simulink model "MPC_resetable_THISONE"  (R2020b)
settings: Solver=VariableStepAuto  StartTime=0.0  StopTime=10  FixedStep=0.01  RelTol=1e-3
values from neighbouring files (symbols this model uses):
  A_2 = zeros(3)    [MPC_tune.m]
  B_2 = I_inv    [MPC_tune.m]
  C_2 = eye(3)    [MPC_tune.m]
  D_2 = zeros(3)    [MPC_tune.m]
  I_inv = inv(I_mat)    [MPC_tune.m]
undefined symbols (not defined in the file or in its folder): theta0
libraries: pid_lib x3, fuzblock x3, mpclib x1, dspmathops x1
settings Model: Creator=Jonathan van Zyl  LastModifiedBy=Jonathan van Zyl

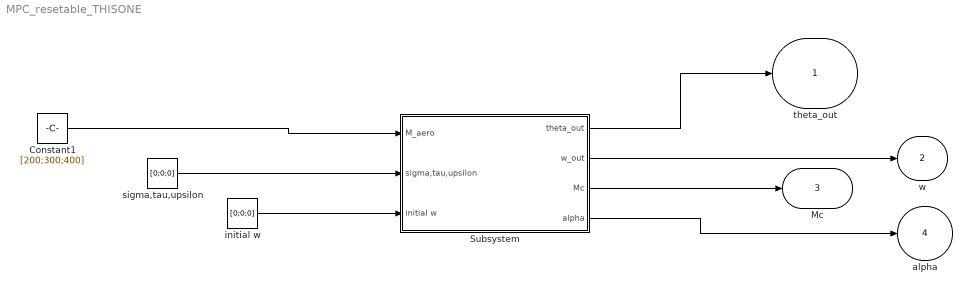
== system MPC_resetable_THISONE ==
  Constant1 : Constant  Value=[200;300;400]
  Subsystem : Subsystem
  initial w : Constant  Value=[0;0;0]
  sigma,tau,upsilon : Constant  Value=[0;0;0]
  theta_out : Outport
  w : Outport  Port=2
  Mc : Outport  Port=3
  alpha : Outport  Port=4
  wires:
  Constant1/1 -> Subsystem/1(M_aero)
  sigma,tau,upsilon/1 -> Subsystem/2(sigma,tau,upsilon)
  initial w/1 -> Subsystem/3(initial w)
  Subsystem/1(theta_out) -> theta_out/1
  Subsystem/2(w_out) -> w/1
  Subsystem/3(Mc) -> Mc/1
  Subsystem/4(alpha) -> alpha/1

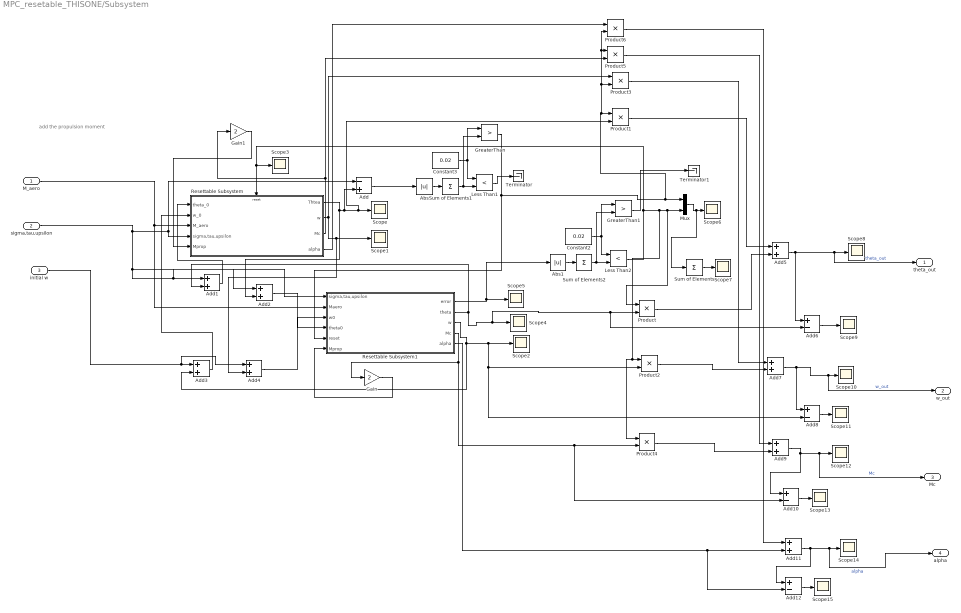
== system MPC_resetable_THISONE/Subsystem ==
  note: add the propulsion moment
  M_aero : Inport
  sigma,tau,upsilon : Inport  Port=2
  initial w : Inport  Port=3
  Abs : Abs
  Abs1 : Abs
  Add : Sum  Inputs=-+
  Add{1..5,7,9,11} (8 alike) : Sum
  Add{6,8,10,12} (4 alike) : Sum  Inputs=+-
  Constant2 : Constant  Value=0.02
  Constant3 : Constant  Value=0.02
  Gain : Gain  Gain=2
  Gain1 : Gain  Gain=2
  GreaterThan : RelationalOperator  Operator=>  OutDataTypeStr=boolean  RndMeth=Simplest
  GreaterThan1 : RelationalOperator  Operator=>  OutDataTypeStr=boolean  RndMeth=Simplest
  Less Than1 : RelationalOperator  Operator=<  OutDataTypeStr=boolean  RndMeth=Simplest
  Less Than2 : RelationalOperator  Operator=<  OutDataTypeStr=boolean  RndMeth=Simplest
  Mux : Mux  Inputs=2
  Product{,1..6} (7 alike) : Product
  Resettable Subsystem : Subsystem  TreatAsAtomicUnit=on
  Resettable Subsystem1 : Subsystem  TreatAsAtomicUnit=on
  Scope{,1..15} (16 alike) : Scope
  Sum of Elements : Sum  Inputs=+
  Sum of Elements1 : Sum  Inputs=+
  Sum of Elements2 : Sum  Inputs=+
  Terminator : Terminator
  Terminator1 : Terminator
  theta_out : Outport
  w_out : Outport  Port=2
  Mc : Outport  Port=3
  alpha : Outport  Port=4
  wires:
  Add8/1 -> Scope11/1
  GreaterThan/1 -> Product6/2, Product5/1, Product3/2, Product1/1, Mux/1, Resettable Subsystem1/5(reset)
  Add6/1 -> Scope9/1
  Abs1/1 -> Sum of Elements2/1
  Product1/1 -> Add5/1
  Resettable Subsystem/2(w) -> Scope1/1, Add4/2, Product3/1
  Resettable Subsystem1/4(Mc) -> Add10/2, Product4/2, Gain/1
  Resettable Subsystem1/2(theta) -> Add6/2, Product/2, Scope4/1, Add1/2
  Resettable Subsystem1/5(alpha) -> Add12/2, Add11/2
  Resettable Subsystem/1(Thtea) -> Add2/2, Add/2, Product1/2, Scope/1
  Less Than2/1 -> Product2/1, Product4/1, Product/1, Mux/2, Scope3/1, Resettable Subsystem/Reset
  M_aero/1 -> Resettable Subsystem1/2(Maero), Resettable Subsystem/3(M_aero)
  Resettable Subsystem1/1(error) -> Abs1/1, Scope5/1
  Add11/1 -> Add12/1, alpha/1, Scope14/1  "alpha"
  Product2/1 -> Add7/2
  Constant2/1 -> GreaterThan1/1, Less Than2/1
  Resettable Subsystem1/3(w) -> Add3/2, Scope2/1, Add8/2, Product2/2
  Product3/1 -> Add7/1
  Add12/1 -> Scope15/1
  Abs/1 -> Sum of Elements1/1
  Add5/1 -> Add6/1, theta_out/1, Scope8/1  "theta_out"
  Add2/1 -> Resettable Subsystem1/4(theta0)
  Constant3/1 -> GreaterThan/1, Less Than1/1
  Sum of Elements1/1 -> Less Than1/2, GreaterThan/2
  Add3/1 -> Resettable Subsystem/2(w_0)
  sigma,tau,upsilon/1 -> Add2/1, Add1/1, Resettable Subsystem1/1(sigma,tau,upsilon), Add/1, Resettable Subsystem/4(sigma,tau,upsilon)
  Product5/1 -> Add9/1
  Resettable Subsystem/3(Mc) -> Product5/2, Gain1/1
  Add7/1 -> Add8/1, w_out/1, Scope10/1  "w_out"
  Product6/1 -> Add11/1
  Add9/1 -> Add10/1, Mc/1, Scope12/1  "Mc"
  Add/1 -> Abs/1
  Add1/1 -> Resettable Subsystem/1(theta_0)
  Sum of Elements/1 -> Scope7/1
  Gain/1 -> Resettable Subsystem1/6(Mprop)
  Sum of Elements2/1 -> Less Than2/2, GreaterThan1/2
  Gain1/1 -> Resettable Subsystem/5(Mprop)
  Mux/1 -> Sum of Elements/1, Scope6/1
  Resettable Subsystem/4(alpha) -> Product6/1
  Add4/1 -> Resettable Subsystem1/3(w0)
  initial w/1 -> Add4/1, Add3/1
  Product/1 -> Add5/2
  Add10/1 -> Scope13/1
  Product4/1 -> Add9/2
  GreaterThan1/1 -> Terminator1/1
  Less Than1/1 -> Terminator/1

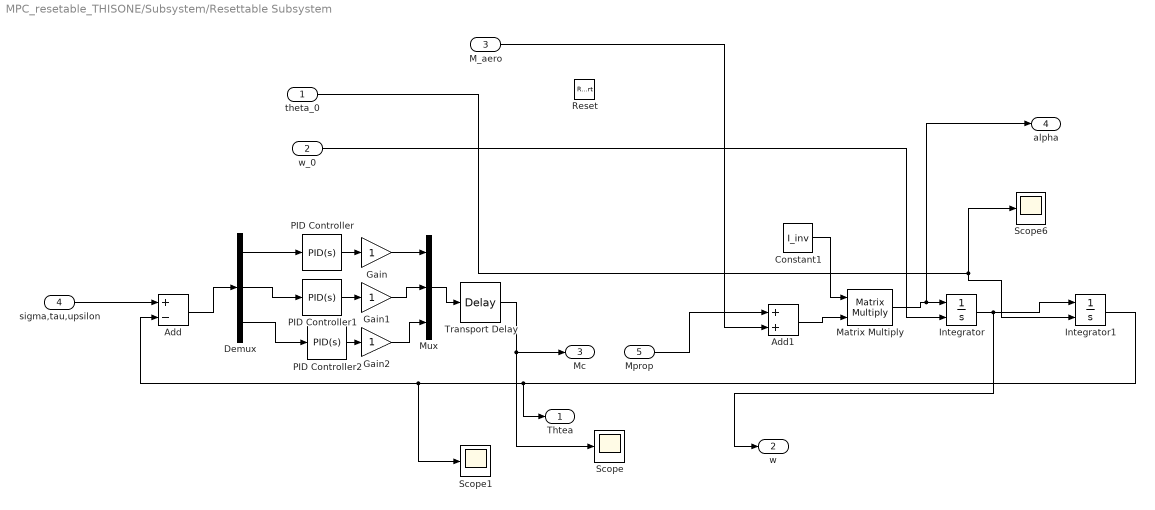
== system MPC_resetable_THISONE/Subsystem/Resettable Subsystem ==
  theta_0 : Inport
  w_0 : Inport  Port=2
  M_aero : Inport  Port=3
  sigma,tau,upsilon : Inport  Port=4
  Mprop : Inport  Port=5
  Reset : ResetPort  DisableCoverage=on  ResetTriggerType=either
  Add : Sum  Inputs=+-
  Add1 : Sum
  Constant1 : Constant  Value=I_inv
  Demux : Demux  Outputs=3
  Gain : Gain
  Gain1 : Gain
  Gain2 : Gain
  Integrator : Integrator  InitialConditionSource=external  InitialCondition=[0.15;-0.2;0.01]
  Integrator1 : Integrator  InitialConditionSource=external  InitialCondition=[0.01;-0.01;0.005]
  Matrix Multiply : Product  Multiplication=Matrix(*)
  Mux : Mux  Inputs=3
  PID Controller : pid_lib/PID Controller  Controller=PID  Form=Parallel  TimeDomain=Continuous-time  UseExternalTs=off  SampleTime=-1  IntegratorMethod=Forward Euler  FilterMethod=Forward Euler  ControllerParametersSource=internal  P=76.4274415550338  I=3.57793373088927  D=400.875615235633  UseFilter=on  N=5.45397025421619  TunerSelectOption=Transfer Function Based (PID Tuner App)  InitialConditionSource=internal  InitialConditionForIntegrator=0  InitialConditionForFilter=0  DifferentiatorICPrevScaledInput=0  ExternalReset=none  TrackingMode=off  Kt=1  LimitOutput=off  SatLimitsSource=internal  UpperSaturationLimit=inf  LowerSaturationLimit=-inf  LinearizeAsGain=on  AntiWindupMode=none  Kb=1  POutMin=[]  POutMax=[]  IOutMin=[]  IOutMax=[]  DOutMin=[]  DOutMax=[]  NOutMin=[]  NOutMax=[]  SumOutMin=[]  SumOutMax=[]  SaturationOutMin=[]  SaturationOutMax=[]  PParamMin=[]  PParamMax=[]  IParamMin=[]  IParamMax=[]  DParamMin=[]  DParamMax=[]  NParamMin=[]  NParamMax=[]  KbParamMin=[]  KbParamMax=[]  KtParamMin=[]  KtParamMax=[]  KbOutMin=[]  KbOutMax=[]  KtOutMin=[]  KtOutMax=[]  IntegratorOutMin=[]  IntegratorOutMax=[]  FilterOutMin=[]  FilterOutMax=[]  SumI1OutMin=[]  SumI1OutMax=[]  SumI2OutMin=[]  SumI2OutMax=[]  SumI3OutMin=[]  SumI3OutMax=[]  SumI4OutMin=[]  SumI4OutMax=[]  SumDOutMin=[]  SumDOutMax=[]  DifferentiatorOutMin=[]  DifferentiatorOutMax=[]  FilterDiffOutCoefMin=[]  FilterDiffOutCoefMax=[]  ReciprocalOutMin=[]  ReciprocalOutMax=[]  SumDenOutMin=[]  SumDenOutMax=[]  SumNumOutMin=[]  SumNumOutMax=[]  DivideOutMin=[]  DivideOutMax=[]  UdiffTsProdOutMin=[]  UdiffTsProdOutMax=[]  NTsProdOutMin=[]  NTsProdOutMax=[]  UintegralTsProdOutMin=[]  UintegralTsProdOutMax=[]  UngainTsProdOutMin=[]  UngainTsProdOutMax=[]  IntegratorContinuousStateAttributes=''  IntegratorStateMustResolveToSignalObject=off  IntegratorRTWStateStorageClass=Auto  FilterContinuousStateAttributes=''  FilterStateMustResolveToSignalObject=off  FilterRTWStateStorageClass=Auto  ParallelPVariant=InternalParameters  IdealPVariant=Disabled  IVariant=InternalParameters  DVariant=InternalParameters  IntegratorVariant=Continuous  SatVariant=Disabled  AWVariant=Passthrough  PCopyVariant=Disabled  TRVariant=Disabled  FdbkBlocksVariant=Forward  IdealPFdbkVariant=Disabled  SatFdbkVariant=Disabled  DerivativeFilterVariant=ContFilter  NVariant=InternalParameters  NCopyVariant=Disabled  FilterICVariant=InternalICsFilter  IntegratorICVariant=InternalICs  ExternalResetVariant=Disabled  TRSumVariant=Passthrough  SumFdbkVariant=Disabled  SumVariant=Sum_PID  TsampFilterVariant=InternalTs  TsampNgainVariant=Passthrough  TsampIntegralVariant=Passthrough  ExternalSaturationOutDataTypeStr=Inherit: Same as second input
  PID Controller1 : pid_lib/PID Controller  Controller=PID  Form=Parallel  TimeDomain=Continuous-time  UseExternalTs=off  SampleTime=-1  IntegratorMethod=Forward Euler  FilterMethod=Forward Euler  ControllerParametersSource=internal  P=-202.527799620363  I=-9.48129403471772  D=-1062.29457146841  UseFilter=on  N=5.45397025421619  TunerSelectOption=Transfer Function Based (PID Tuner App)  InitialConditionSource=internal  InitialConditionForIntegrator=0  InitialConditionForFilter=0  DifferentiatorICPrevScaledInput=0  ExternalReset=none  TrackingMode=off  Kt=1  LimitOutput=off  SatLimitsSource=internal  UpperSaturationLimit=inf  LowerSaturationLimit=-inf  LinearizeAsGain=on  AntiWindupMode=none  Kb=1  POutMin=[]  POutMax=[]  IOutMin=[]  IOutMax=[]  DOutMin=[]  DOutMax=[]  NOutMin=[]  NOutMax=[]  SumOutMin=[]  SumOutMax=[]  SaturationOutMin=[]  SaturationOutMax=[]  PParamMin=[]  PParamMax=[]  IParamMin=[]  IParamMax=[]  DParamMin=[]  DParamMax=[]  NParamMin=[]  NParamMax=[]  KbParamMin=[]  KbParamMax=[]  KtParamMin=[]  KtParamMax=[]  KbOutMin=[]  KbOutMax=[]  KtOutMin=[]  KtOutMax=[]  IntegratorOutMin=[]  IntegratorOutMax=[]  FilterOutMin=[]  FilterOutMax=[]  SumI1OutMin=[]  SumI1OutMax=[]  SumI2OutMin=[]  SumI2OutMax=[]  SumI3OutMin=[]  SumI3OutMax=[]  SumI4OutMin=[]  SumI4OutMax=[]  SumDOutMin=[]  SumDOutMax=[]  DifferentiatorOutMin=[]  DifferentiatorOutMax=[]  FilterDiffOutCoefMin=[]  FilterDiffOutCoefMax=[]  ReciprocalOutMin=[]  ReciprocalOutMax=[]  SumDenOutMin=[]  SumDenOutMax=[]  SumNumOutMin=[]  SumNumOutMax=[]  DivideOutMin=[]  DivideOutMax=[]  UdiffTsProdOutMin=[]  UdiffTsProdOutMax=[]  NTsProdOutMin=[]  NTsProdOutMax=[]  UintegralTsProdOutMin=[]  UintegralTsProdOutMax=[]  UngainTsProdOutMin=[]  UngainTsProdOutMax=[]  IntegratorContinuousStateAttributes=''  IntegratorStateMustResolveToSignalObject=off  IntegratorRTWStateStorageClass=Auto  FilterContinuousStateAttributes=''  FilterStateMustResolveToSignalObject=off  FilterRTWStateStorageClass=Auto  ParallelPVariant=InternalParameters  IdealPVariant=Disabled  IVariant=InternalParameters  DVariant=InternalParameters  IntegratorVariant=Continuous  SatVariant=Disabled  AWVariant=Passthrough  PCopyVariant=Disabled  TRVariant=Disabled  FdbkBlocksVariant=Forward  IdealPFdbkVariant=Disabled  SatFdbkVariant=Disabled  DerivativeFilterVariant=ContFilter  NVariant=InternalParameters  NCopyVariant=Disabled  FilterICVariant=InternalICsFilter  IntegratorICVariant=InternalICs  ExternalResetVariant=Disabled  TRSumVariant=Passthrough  SumFdbkVariant=Disabled  SumVariant=Sum_PID  TsampFilterVariant=InternalTs  TsampNgainVariant=Passthrough  TsampIntegralVariant=Passthrough  ExternalSaturationOutDataTypeStr=Inherit: Same as second input
  PID Controller2 : pid_lib/PID Controller  Controller=PID  Form=Parallel  TimeDomain=Continuous-time  UseExternalTs=off  SampleTime=-1  IntegratorMethod=Forward Euler  FilterMethod=Forward Euler  ControllerParametersSource=internal  P=-232.294042315359  I=-10.8747940867059  D=-1218.42384402842  UseFilter=on  N=5.45397025421619  TunerSelectOption=Transfer Function Based (PID Tuner App)  InitialConditionSource=internal  InitialConditionForIntegrator=0  InitialConditionForFilter=0  DifferentiatorICPrevScaledInput=0  ExternalReset=none  TrackingMode=off  Kt=1  LimitOutput=off  SatLimitsSource=internal  UpperSaturationLimit=inf  LowerSaturationLimit=-inf  LinearizeAsGain=on  AntiWindupMode=none  Kb=1  POutMin=[]  POutMax=[]  IOutMin=[]  IOutMax=[]  DOutMin=[]  DOutMax=[]  NOutMin=[]  NOutMax=[]  SumOutMin=[]  SumOutMax=[]  SaturationOutMin=[]  SaturationOutMax=[]  PParamMin=[]  PParamMax=[]  IParamMin=[]  IParamMax=[]  DParamMin=[]  DParamMax=[]  NParamMin=[]  NParamMax=[]  KbParamMin=[]  KbParamMax=[]  KtParamMin=[]  KtParamMax=[]  KbOutMin=[]  KbOutMax=[]  KtOutMin=[]  KtOutMax=[]  IntegratorOutMin=[]  IntegratorOutMax=[]  FilterOutMin=[]  FilterOutMax=[]  SumI1OutMin=[]  SumI1OutMax=[]  SumI2OutMin=[]  SumI2OutMax=[]  SumI3OutMin=[]  SumI3OutMax=[]  SumI4OutMin=[]  SumI4OutMax=[]  SumDOutMin=[]  SumDOutMax=[]  DifferentiatorOutMin=[]  DifferentiatorOutMax=[]  FilterDiffOutCoefMin=[]  FilterDiffOutCoefMax=[]  ReciprocalOutMin=[]  ReciprocalOutMax=[]  SumDenOutMin=[]  SumDenOutMax=[]  SumNumOutMin=[]  SumNumOutMax=[]  DivideOutMin=[]  DivideOutMax=[]  UdiffTsProdOutMin=[]  UdiffTsProdOutMax=[]  NTsProdOutMin=[]  NTsProdOutMax=[]  UintegralTsProdOutMin=[]  UintegralTsProdOutMax=[]  UngainTsProdOutMin=[]  UngainTsProdOutMax=[]  IntegratorContinuousStateAttributes=''  IntegratorStateMustResolveToSignalObject=off  IntegratorRTWStateStorageClass=Auto  FilterContinuousStateAttributes=''  FilterStateMustResolveToSignalObject=off  FilterRTWStateStorageClass=Auto  ParallelPVariant=InternalParameters  IdealPVariant=Disabled  IVariant=InternalParameters  DVariant=InternalParameters  IntegratorVariant=Continuous  SatVariant=Disabled  AWVariant=Passthrough  PCopyVariant=Disabled  TRVariant=Disabled  FdbkBlocksVariant=Forward  IdealPFdbkVariant=Disabled  SatFdbkVariant=Disabled  DerivativeFilterVariant=ContFilter  NVariant=InternalParameters  NCopyVariant=Disabled  FilterICVariant=InternalICsFilter  IntegratorICVariant=InternalICs  ExternalResetVariant=Disabled  TRSumVariant=Passthrough  SumFdbkVariant=Disabled  SumVariant=Sum_PID  TsampFilterVariant=InternalTs  TsampNgainVariant=Passthrough  TsampIntegralVariant=Passthrough  ExternalSaturationOutDataTypeStr=Inherit: Same as second input
  Scope : Scope
  Scope1 : Scope
  Scope6 : Scope
  Transport Delay : TransportDelay  DelayTime=0.1
  Thtea : Outport
  w : Outport  Port=2
  Mc : Outport  Port=3
  alpha : Outport  Port=4
  wires:
  Transport Delay/1 -> Mc/1, Scope/1
  Constant1/1 -> Matrix Multiply/1
  PID Controller2/1 -> Gain2/1
  PID Controller/1 -> Gain/1
  Matrix Multiply/1 -> alpha/1, Integrator/1
  Demux/3 -> PID Controller2/1
  Mux/1 -> Transport Delay/1
  sigma,tau,upsilon/1 -> Add/1
  Gain/1 -> Mux/1
  w_0/1 -> Integrator/2
  Gain2/1 -> Mux/3
  Add/1 -> Demux/1
  Add1/1 -> Matrix Multiply/2
  PID Controller1/1 -> Gain1/1
  Integrator/1 -> w/1, Integrator1/1
  theta_0/1 -> Integrator1/2, Scope6/1
  Demux/2 -> PID Controller1/1
  Gain1/1 -> Mux/2
  M_aero/1 -> Add1/2
  Demux/1 -> PID Controller/1
  Integrator1/1 -> Thtea/1, Scope1/1, Add/2
  Mprop/1 -> Add1/1

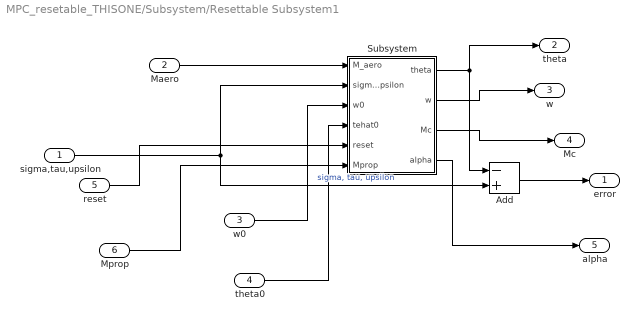
== system MPC_resetable_THISONE/Subsystem/Resettable Subsystem1 ==
  sigma,tau,upsilon : Inport
  Maero : Inport  Port=2
  w0 : Inport  Port=3
  theta0 : Inport  Port=4
  reset : Inport  Port=5
  Mprop : Inport  Port=6
  Add : Sum  Inputs=-+
  Subsystem : Subsystem
  error : Outport
  theta : Outport  Port=2
  w : Outport  Port=3
  Mc : Outport  Port=4
  alpha : Outport  Port=5
  wires:
  theta0/1 -> Subsystem/4(tehat0)
  Subsystem/2(w) -> w/1
  Add/1 -> error/1
  Maero/1 -> Subsystem/1(M_aero)
  sigma,tau,upsilon/1 -> Add/2, Subsystem/2(sigma,tau,upsilon)  "sigma, tau, upsilon"
  Subsystem/1(theta) -> Add/1, theta/1
  w0/1 -> Subsystem/3(w0)
  reset/1 -> Subsystem/5(reset)
  Subsystem/3(Mc) -> Mc/1
  Mprop/1 -> Subsystem/6(Mprop)
  Subsystem/4(alpha) -> alpha/1

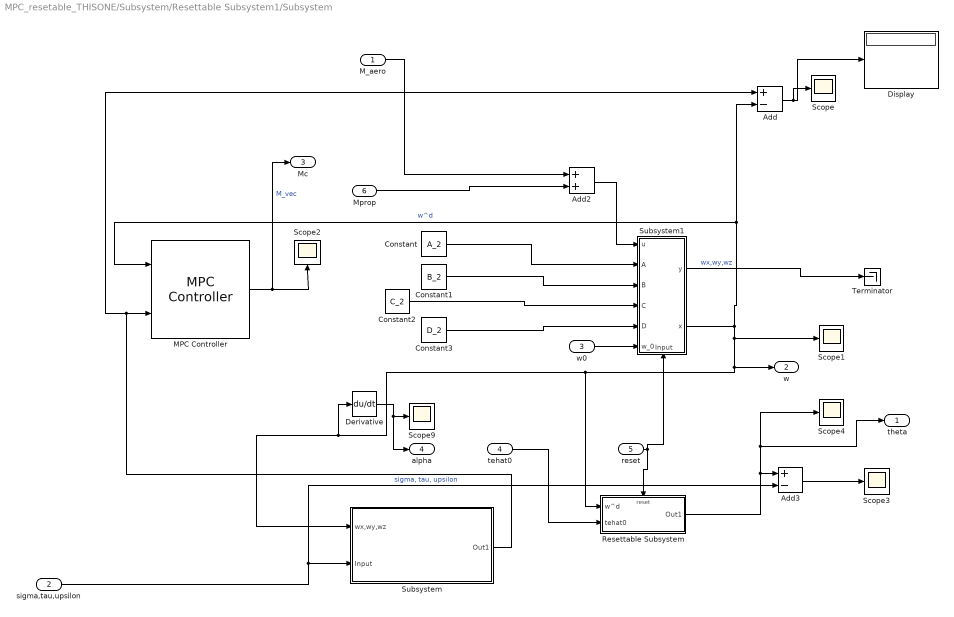
== system MPC_resetable_THISONE/Subsystem/Resettable Subsystem1/Subsystem ==
  M_aero : Inport
  sigma,tau,upsilon : Inport  Port=2
  w0 : Inport  Port=3
  tehat0 : Inport  Port=4
  reset : Inport  Port=5
  Mprop : Inport  Port=6
  Add : Sum  Inputs=+-
  Add2 : Sum
  Add3 : Sum  Inputs=+-
  Constant : Constant  Value=A_2
  Constant1 : Constant  Value=B_2
  Constant2 : Constant  Value=C_2
  Constant3 : Constant  Value=D_2
  Derivative : Derivative
  Display : Display
  MPC Controller : mpclib/MPC Controller  SCDEnableBlockLinearizationSpecification=on  mpcobj=MPCDesignerSession.AppData.Controllers.MPC  is_multiple=0  enable_value=0  return_u0=off  updateMPCinCallerWorkspace=on  md_inport=off  mv_inport=off  uref_inport=off  return_cost=off  return_mvseq=off  return_qpstatus=off  return_xseq=off  return_state=off  return_ovseq=off  state_inport=off  umin_inport=off  umax_inport=off  ymin_inport=off  ymax_inport=off  cc_inport=off  ywt_inport=off  uwt_inport=off  duwt_inport=off  rhoeps_inport=off  pm_inport=off  MaximumP=10  HorizonChoice=FixedHorizon  n_ts=0.1  n_p=10  n_mv=3  n_md=0  n_ud=0  n_mo=3  n_uo=0  BlockDataType=double  SampleTimeInherited=off  switch_inport=off
  Resettable Subsystem : Subsystem  TreatAsAtomicUnit=on
  Scope{,1..4,9} (6 alike) : Scope
  Subsystem : Subsystem
  Subsystem1 : Subsystem
      settings: PortSchema="{\"entries\":[{\"content\":{\"sides\":[{\"content\":{\"connectorIds\":[\"In1\",\"In2\",\"In3\",\"In4\",\"In5\",\"In6\"]},\"type\":\"ConnectorPlacement.EquallySpacedRectSide\",\"uuid\":\"7d9460a7-3adf-4f89-91e7-b456f7078c86\"},{\"content\":{\"connectorIds\":[\"Out1\",\"Out2\"],\"side\":\"RIGHT\"},\"type\":\"ConnectorPlacement.EquallySpacedRectSide\",\"uuid\":\"f1bf29ac-ed67-4ce4-91e2-85f2b90efa08\"},{\"content\":{\"connectorIds\":[],\"side\":\"TOP\"},\"type\":\"ConnectorPlacement.EquallySpacedRectSide\",\"uuid\":\"d922c634-a6d8-424b-a167-3b858780e5fe\"},{\"content\":{\"connectorIds\":[\"In7\"],\"side\":\"BOTTOM\"},\"type\":\"ConnectorPlacement.EquallySpacedRectSide\",\"uuid\":\"f177f641-1570-409d-a38e-cef2b78f705f\"},{\"content\":{\"connectorIds\":[],\"side\":\"HIDDEN\"},\"type\":\"ConnectorPlacement.EquallySpacedRectSide\",\"uuid\":\"30cf80c6-7b26-40df-a778-919a6a544dd2\"}]},\"type\":\"ConnectorPlacement.EquallySpacedConnector\",\"uuid\":\"27252b95-3211-4624-87a6-4be9d32d6c6a\"}],\"packageUris\":[\"http://schema.mathworks.com/mf0/Connector/R2020b\"],\"version\":\"1.0\"}"
  Terminator : Terminator
  theta : Outport
  w : Outport  Port=2
  Mc : Outport  Port=3
  alpha : Outport  Port=4
  wires:
  Subsystem1/1(y) -> Terminator/1  "wx,wy,wz"
  Derivative/1 -> alpha/1, Scope9/1
  Resettable Subsystem/1(Out1) -> Scope4/1, theta/1, Add3/1
  Add/1 -> Display/1, Scope/1
  Add3/1 -> Scope3/1
  Add2/1 -> Subsystem1/1(u)
  sigma,tau,upsilon/1 -> Add3/2, Subsystem/2(Input)  "sigma, tau, upsilon"
  Subsystem/1(Out1) -> Add/1, MPC Controller/2
  M_aero/1 -> Add2/1
  Constant2/1 -> Subsystem1/4(C)
  Constant3/1 -> Subsystem1/5(D)
  Subsystem1/2(x) -> Add/2, MPC Controller/1, Scope1/1, w/1, Resettable Subsystem/1(w^d), Subsystem/1(wx,wy,wz), Derivative/1  "w^d"
  MPC Controller/1 -> Mc/1, Scope2/1  "M_vec"
  Constant/1 -> Subsystem1/2(A)
  Constant1/1 -> Subsystem1/3(B)
  w0/1 -> Subsystem1/6(w_0)
  tehat0/1 -> Resettable Subsystem/2(tehat0)
  reset/1 -> Subsystem1/7(Input), Resettable Subsystem/Reset
  Mprop/1 -> Add2/2

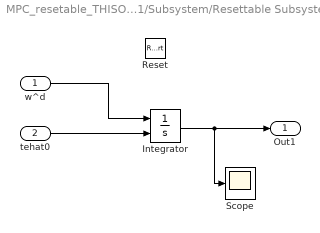
== system MPC_resetable_THISONE/Subsystem/Resettable Subsystem1/Subsystem/Resettable Subsystem ==
  w^d : Inport
  tehat0 : Inport  Port=2
  Reset : ResetPort  DisableCoverage=on
  Integrator : Integrator  InitialConditionSource=external  InitialCondition=theta0
  Scope : Scope
  Out1 : Outport
  wires:
  tehat0/1 -> Integrator/2
  w^d/1 -> Integrator/1
  Integrator/1 -> Scope/1, Out1/1

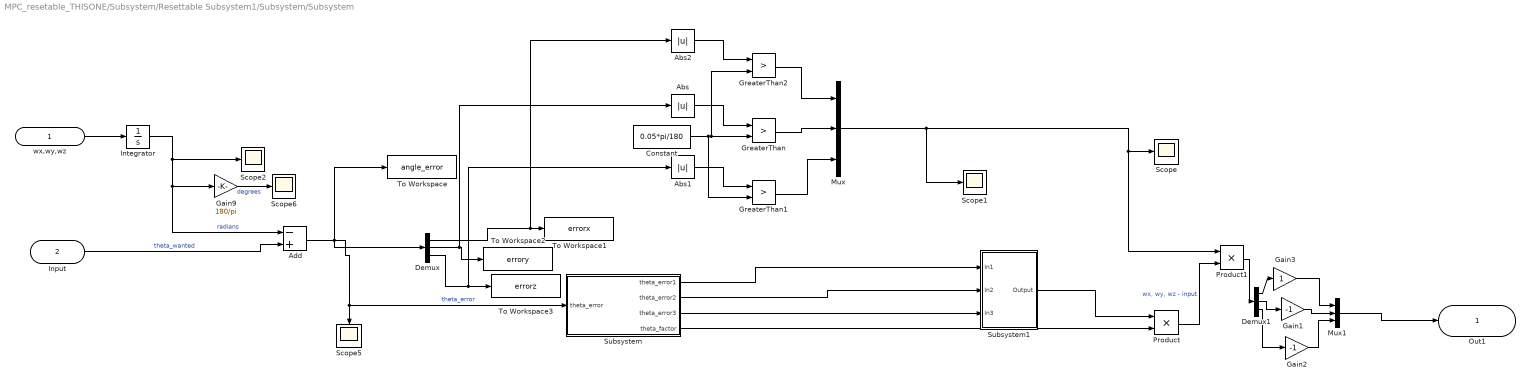
== system MPC_resetable_THISONE/Subsystem/Resettable Subsystem1/Subsystem/Subsystem ==
  wx,wy,wz : Inport
  Input : Inport  Port=2
  Abs : Abs
  Abs1 : Abs
  Abs2 : Abs
  Add : Sum  Inputs=-+
  Constant : Constant  Value=0.05*pi/180
  Demux : Demux  Outputs=3
  Demux1 : Demux  Outputs=3
  Gain1 : Gain  Gain=-1
  Gain2 : Gain  Gain=-1
  Gain3 : Gain
  Gain9 : Gain  Gain=180/pi
  GreaterThan : RelationalOperator  Operator=>  OutDataTypeStr=boolean  RndMeth=Simplest
  GreaterThan1 : RelationalOperator  Operator=>  OutDataTypeStr=boolean  RndMeth=Simplest
  GreaterThan2 : RelationalOperator  Operator=>  OutDataTypeStr=boolean  RndMeth=Simplest
  Integrator : Integrator  InitialCondition=[0;0;0]
  Mux : Mux  Inputs=3
  Mux1 : Mux  Inputs=3
  Product : Product
  Product1 : Product
  Scope{,1..2,5..6} (5 alike) : Scope
  Subsystem : Subsystem
  Subsystem1 : Subsystem
  To Workspace : ToWorkspace  VariableName=angle_error  SampleTime=-1
  To Workspace1 : ToWorkspace  VariableName=errorx  SaveFormat=Timeseries  SampleTime=-1
      settings: Save2DSignal=2-D array (concatenate along first dimension)
  To Workspace2 : ToWorkspace  VariableName=errory  SaveFormat=Timeseries  SampleTime=-1
  To Workspace3 : ToWorkspace  VariableName=errorz  SaveFormat=Timeseries  SampleTime=-1
  Out1 : Outport
  wires:
  Integrator/1 -> Add/1, Gain9/1, Scope2/1  "radians"
  Add/1 -> To Workspace/1, Demux/1, Subsystem/1(theta_error), Scope5/1  "theta_error"
  Gain9/1 -> Scope6/1  "degrees"
  Input/1 -> Add/2  "theta_wanted"
  Product/1 -> Product1/2  "wx, wy, wz - input"
  wx,wy,wz/1 -> Integrator/1
  Subsystem/4(theta_factor) -> Product/2
  Demux/2 -> Abs/1, To Workspace2/1
  Demux/3 -> Abs1/1, To Workspace3/1
  Demux/1 -> Abs2/1, To Workspace1/1
  Subsystem/1(theta_error1) -> Subsystem1/1(In1)
  Subsystem/2(theta_error2) -> Subsystem1/2(In2)
  Subsystem/3(theta_error3) -> Subsystem1/3(In3)
  Subsystem1/1(Output) -> Product/1
  Abs/1 -> GreaterThan/1
  Constant/1 -> GreaterThan1/2, GreaterThan2/2, GreaterThan/2
  Abs1/1 -> GreaterThan1/1
  Abs2/1 -> GreaterThan2/1
  GreaterThan2/1 -> Mux/1
  GreaterThan/1 -> Mux/2
  GreaterThan1/1 -> Mux/3
  Mux/1 -> Scope1/1, Scope/1, Product1/1
  Product1/1 -> Demux1/1
  Mux1/1 -> Out1/1
  Demux1/2 -> Gain1/1
  Demux1/3 -> Gain2/1
  Demux1/1 -> Gain3/1
  Gain3/1 -> Mux1/1
  Gain1/1 -> Mux1/2
  Gain2/1 -> Mux1/3

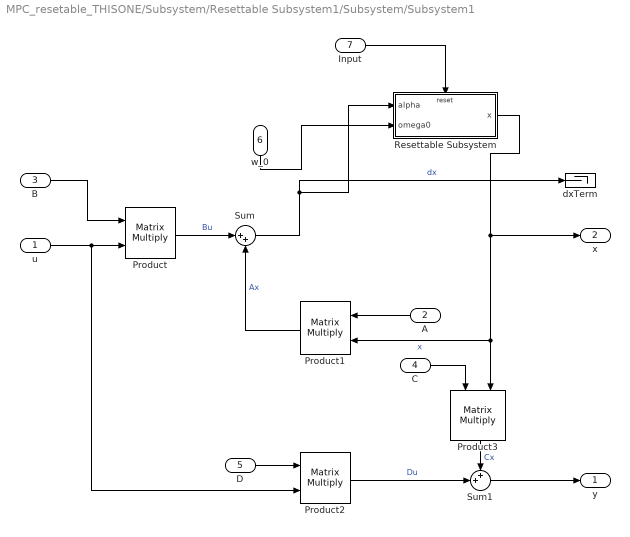
== system MPC_resetable_THISONE/Subsystem/Resettable Subsystem1/Subsystem/Subsystem1 ==
  u : Inport
  A : Inport  Port=2
  B : Inport  Port=3
  C : Inport  Port=4
  D : Inport  Port=5
  w_0 : Inport  Port=6
  Input : Inport  Port=7
  Product{,1..3} (4 alike) : Product  SCDEnableBlockLinearizationSpecification=on  Multiplication=Matrix(*)
  Resettable Subsystem : Subsystem  TreatAsAtomicUnit=on
  Sum : Sum  Inputs=|++
  Sum1 : Sum  Inputs=++|
  dxTerm : Terminator
  y : Outport  VectorParamsAs1DForOutWhenUnconnected=off
  x : Outport  Port=2  VectorParamsAs1DForOutWhenUnconnected=off
  wires:
  Sum/1 -> Resettable Subsystem/1(alpha), dxTerm/1  "dx"
  Product3/1 -> Sum1/1  "Cx"
  Product/1 -> Sum/1  "Bu"
  u/1 -> Product2/2, Product/2
  Product2/1 -> Sum1/2  "Du"
  Resettable Subsystem/1(x) -> x/1, Product1/2, Product3/2  "x"
  A/1 -> Product1/1
  Product1/1 -> Sum/2  "Ax"
  C/1 -> Product3/1
  B/1 -> Product/1
  D/1 -> Product2/1
  Sum1/1 -> y/1
  w_0/1 -> Resettable Subsystem/2(omega0)
  Input/1 -> Resettable Subsystem/Reset

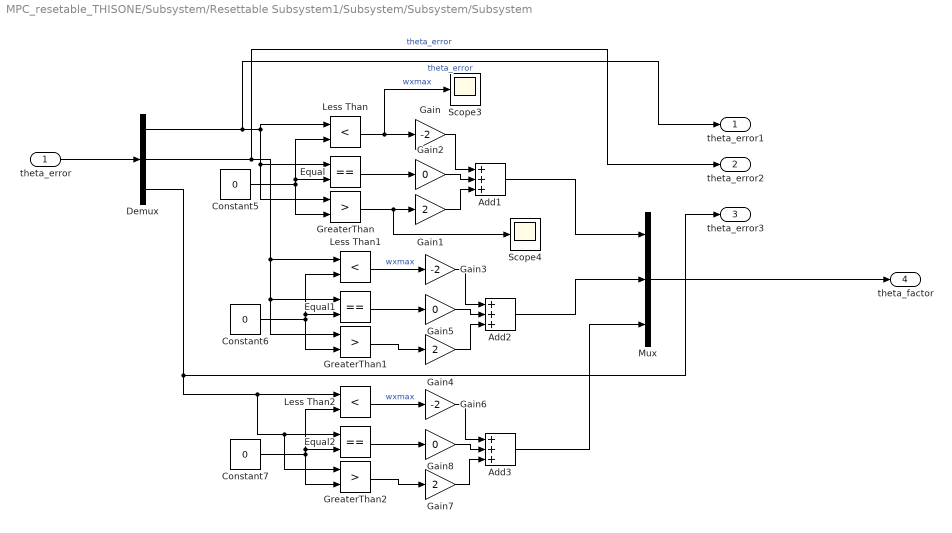
== system MPC_resetable_THISONE/Subsystem/Resettable Subsystem1/Subsystem/Subsystem/Subsystem ==
  theta_error : Inport
  Add1 : Sum  Inputs=+++
  Add2 : Sum  Inputs=+++
  Add3 : Sum  Inputs=+++
  Constant5 : Constant  Value=0
  Constant6 : Constant  Value=0
  Constant7 : Constant  Value=0
  Demux : Demux  Outputs=3
  Equal : RelationalOperator  Operator===  OutDataTypeStr=boolean  RndMeth=Simplest
  Equal1 : RelationalOperator  Operator===  OutDataTypeStr=boolean  RndMeth=Simplest
  Equal2 : RelationalOperator  Operator===  OutDataTypeStr=boolean  RndMeth=Simplest
  Gain : Gain  Gain=-2
  Gain1 : Gain  Gain=2
  Gain2 : Gain  Gain=0
  Gain3 : Gain  Gain=-2
  Gain4 : Gain  Gain=2
  Gain5 : Gain  Gain=0
  Gain6 : Gain  Gain=-2
  Gain7 : Gain  Gain=2
  Gain8 : Gain  Gain=0
  GreaterThan : RelationalOperator  Operator=>  OutDataTypeStr=boolean  RndMeth=Simplest
  GreaterThan1 : RelationalOperator  Operator=>  OutDataTypeStr=boolean  RndMeth=Simplest
  GreaterThan2 : RelationalOperator  Operator=>  OutDataTypeStr=boolean  RndMeth=Simplest
  Less Than : RelationalOperator  Operator=<  OutDataTypeStr=boolean  RndMeth=Simplest
  Less Than1 : RelationalOperator  Operator=<  OutDataTypeStr=boolean  RndMeth=Simplest
  Less Than2 : RelationalOperator  Operator=<  OutDataTypeStr=boolean  RndMeth=Simplest
  Mux : Mux  Inputs=3
  Scope3 : Scope
  Scope4 : Scope
  theta_error1 : Outport
  theta_error2 : Outport  Port=2
  theta_error3 : Outport  Port=3
  theta_factor : Outport  Port=4
  wires:
  Add1/1 -> Mux/1
  Constant5/1 -> Equal/2, Less Than/2, GreaterThan/2
  Equal2/1 -> Gain8/1
  Demux/1 -> theta_error1/1, GreaterThan/1, Equal/1, Less Than/1  "theta_error"
  GreaterThan2/1 -> Gain7/1
  Gain1/1 -> Add1/3
  Gain7/1 -> Add3/3
  Less Than1/1 -> Gain3/1  "wxmax"
  Gain6/1 -> Add3/1
  Equal/1 -> Gain2/1
  Gain5/1 -> Add2/2
  Add3/1 -> Mux/3
  GreaterThan/1 -> Scope4/1, Gain1/1
  Constant6/1 -> Equal1/2, Less Than1/2, GreaterThan1/2
  Demux/3 -> theta_error3/1, GreaterThan2/1, Equal2/1, Less Than2/1
  Gain3/1 -> Add2/1
  Constant7/1 -> Equal2/2, Less Than2/2, GreaterThan2/2
  Equal1/1 -> Gain5/1
  Gain8/1 -> Add3/2
  Gain4/1 -> Add2/3
  GreaterThan1/1 -> Gain4/1
  Gain/1 -> Add1/1
  Demux/2 -> theta_error2/1, GreaterThan1/1, Equal1/1, Less Than1/1  "theta_error"
  Gain2/1 -> Add1/2
  Add2/1 -> Mux/2
  Less Than/1 -> Scope3/1, Gain/1  "wxmax"
  Less Than2/1 -> Gain6/1  "wxmax"
  theta_error/1 -> Demux/1
  Mux/1 -> theta_factor/1

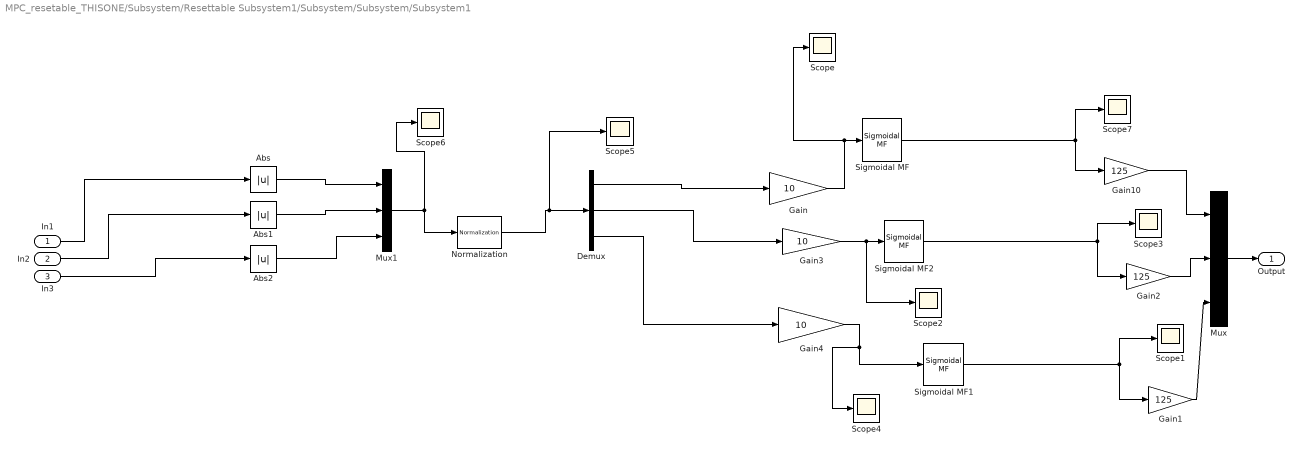
== system MPC_resetable_THISONE/Subsystem/Resettable Subsystem1/Subsystem/Subsystem/Subsystem1 ==
  In1 : Inport
  In2 : Inport  Port=2
  In3 : Inport  Port=3
  Abs : Abs
  Abs1 : Abs
  Abs2 : Abs
  Demux : Demux  Outputs=3
  Gain : Gain  Gain=10
  Gain1 : Gain  Gain=125
  Gain10 : Gain  Gain=125
  Gain2 : Gain  Gain=125
  Gain3 : Gain  Gain=10
  Gain4 : Gain  Gain=10
  Mux : Mux  Inputs=3
  Mux1 : Mux  Inputs=3
  Normalization : dspmathops/Normalization  NormType=Squared 2-norm  Bias=1e-10  NormOver=Each column  Dimension=1  roundingMode=Floor  overflowMode=off  accumDataTypeStr=Inherit: Same as product output  accumLastDataTypeStr=Inherit: Same as product output  outputDataTypeStr=Inherit: Same as product output  outputMin=[]  outputMax=[]  outputLastDataTypeStr=Inherit: Same as product output
  Scope{,1..7} (8 alike) : Scope
  Sigmoidal MF : fuzblock/Membership  Functions/Sigmoidal MF  a=10^(-8)  c=1000
      settings: SourceProductBaseCode=FL
  Sigmoidal MF1 : fuzblock/Membership  Functions/Sigmoidal MF  a=10^(-8)  c=1000
      settings: SourceProductBaseCode=FL
  Sigmoidal MF2 : fuzblock/Membership  Functions/Sigmoidal MF  a=10^(-8)  c=1000
      settings: SourceProductBaseCode=FL
  Output : Outport
  wires:
  Gain2/1 -> Mux/2
  Gain10/1 -> Mux/1
  Sigmoidal MF1/1 -> Gain1/1, Scope1/1
  Sigmoidal MF/1 -> Gain10/1, Scope7/1
  Sigmoidal MF2/1 -> Gain2/1, Scope3/1
  Gain/1 -> Scope/1, Sigmoidal MF/1
  Gain1/1 -> Mux/3
  Gain3/1 -> Scope2/1, Sigmoidal MF2/1
  In2/1 -> Abs1/1
  In1/1 -> Abs/1
  In3/1 -> Abs2/1
  Mux/1 -> Output/1
  Abs/1 -> Mux1/1
  Abs1/1 -> Mux1/2
  Gain4/1 -> Scope4/1, Sigmoidal MF1/1
  Abs2/1 -> Mux1/3
  Demux/3 -> Gain4/1
  Demux/1 -> Gain/1
  Demux/2 -> Gain3/1
  Mux1/1 -> Normalization/1, Scope6/1
  Normalization/1 -> Scope5/1, Demux/1

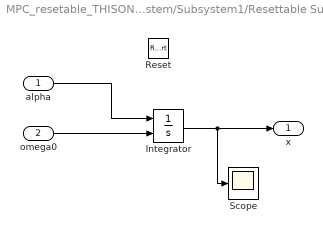
== system MPC_resetable_THISONE/Subsystem/Resettable Subsystem1/Subsystem/Subsystem1/Resettable Subsystem ==
  alpha : Inport
  omega0 : Inport  Port=2
  Reset : ResetPort  DisableCoverage=on
  Integrator : Integrator  InitialConditionSource=external  InitialCondition=theta0
  Scope : Scope
  x : Outport
  wires:
  omega0/1 -> Integrator/2
  alpha/1 -> Integrator/1
  Integrator/1 -> Scope/1, x/1
